simulink model "q_aero_free_osc_response_yaw"  (R2014a)
settings: Solver=ode1  StartTime=0.0  StopTime=5  FixedStep=0.002  RelTol=1e-3
libraries: quarc_library x2, quanser_aero x1
settings Model: SimulationMode=external  ExtModeTrigDuration=5000  Creator=MLevis  LastModifiedBy=MLevis
settings SolverCC: PositivePriorityOrder=on
settings DebuggingCC: MergeDetectMultiDrivingBlocksExec=error
settings RTWCC: SystemTargetFile=quarc_win64.tlc  TemplateMakefile=quarc_default_tmf  Description=QUARC Win64 Target  ProcessScript=quarc_win64_make_rtw_hook
settings GRTTargetCC: ParMdlRefBuildCompliant=off  CompOptLevelCompliant=off  CombineOutputUpdateFcns=off  MatFileLogging=off  CPPClassGenCompliant=off  GRTInterface=on  ExtMode=on  ExtModeMexFile=quarc_comm

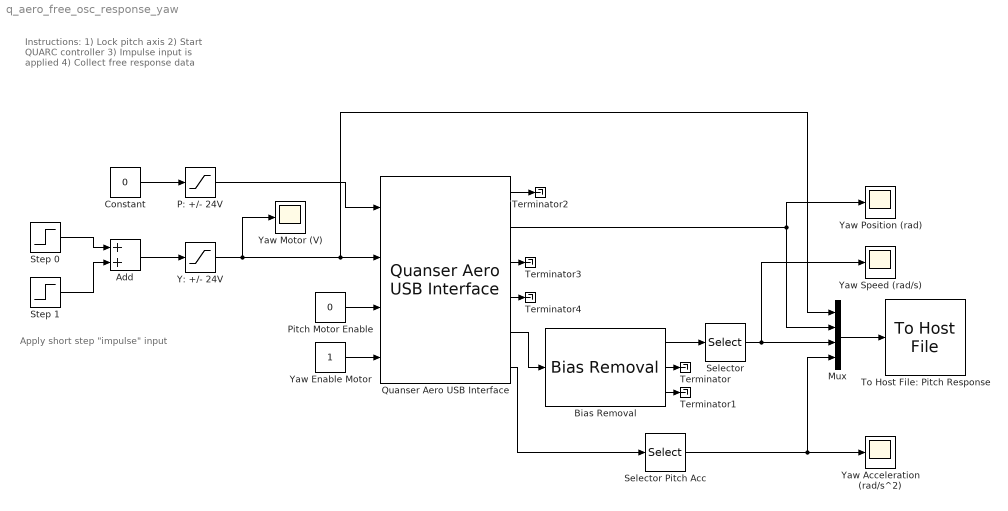
== system q_aero_free_osc_response_yaw ==
  note: Apply short step "impulse" input
  note: Instructions:
      | 1) Lock pitch axis
      | 2) Start QUARC controller
      | 3) Impulse input is applied
      | 4) Collect free response data
  Add : Sum
  Bias Removal : quarc_library/Discrete/Bias Removal  start_time=0  end_time=1  switch_id=0  sample_time=qc_get_step_size
  Constant : Constant  Value=0
  Mux : Mux
  P: +/- 24V : Saturate  UpperLimit=24  LowerLimit=-24
  Pitch Motor Enable : Constant  Value=0
  Quanser Aero USB Interface : quanser_aero/Quanser Aero USB Interface
  Selector : Selector  InputPortWidth=3  Indices=[3]
  Selector Pitch Acc : Selector  InputPortWidth=3  Indices=[3]
  Step 0 : Step  After=20  SampleTime=0
  Step 1 : Step  Time=2  After=-20  SampleTime=0
  Terminator{,1..4} (5 alike) : Terminator
  To Host File: Pitch Response : quarc_library/Sinks/To Host/To Host File  file_name=aero_yaw_free_osc_rsp.mat  variable_name=free_osc_rsp_yaw  decimation=1  sample_time=-1  file_format=MAT-file v.4  options=No header or footer  append=off  final_file_name=aero_yaw_free_osc_rsp.mat
  Y: +/- 24V : Saturate  UpperLimit=24  LowerLimit=-24
  Yaw Acceleration (rad/s^2) : Scope
      settings: TimeRange=10  YMin=-6  YMax=6  SaveName=pitch_spd1
  Yaw Enable Motor : Constant
  Yaw Motor (V) : Scope
      settings: TimeRange=5  YMin=-25  YMax=25  SaveName=ScopeData5
  Yaw Position (rad) : Scope
      settings: TimeRange=5  YMin=-0.5  YMax=1.5  SaveName=ScopeData4
  Yaw Speed (rad/s) : Scope
      settings: TimeRange=5  YMin=-1.5  YMax=1.5  SaveName=pitch_spd
  wires:
  Pitch Motor Enable/1 -> Quanser Aero USB Interface/3
  Yaw Enable Motor/1 -> Quanser Aero USB Interface/4
  Y: +/- 24V/1 -> Quanser Aero USB Interface/2, Mux/1, Yaw Motor (V)/1
  P: +/- 24V/1 -> Quanser Aero USB Interface/1
  Quanser Aero USB Interface/2 -> Mux/2, Yaw Position (rad)/1
  Mux/1 -> To Host File: Pitch Response/1
  Quanser Aero USB Interface/3 -> Terminator3/1
  Quanser Aero USB Interface/4 -> Terminator4/1
  Selector Pitch Acc/1 -> Yaw Acceleration (rad/s^2)/1, Mux/4
  Quanser Aero USB Interface/6 -> Selector Pitch Acc/1
  Step 0/1 -> Add/1
  Step 1/1 -> Add/2
  Add/1 -> Y: +/- 24V/1
  Constant/1 -> P: +/- 24V/1
  Quanser Aero USB Interface/1 -> Terminator2/1
  Bias Removal/2 -> Terminator/1
  Bias Removal/3 -> Terminator1/1
  Bias Removal/1 -> Selector/1
  Quanser Aero USB Interface/5 -> Bias Removal/1
  Selector/1 -> Yaw Speed (rad/s)/1, Mux/3
